simulink model "MotorPositionCntrl"  (R2020a)
settings: Solver=VariableStepAuto  StartTime=0.0  StopTime=10.0  FixedStep=0.01  RelTol=1e-3
undefined symbols (not defined in the file): b, J, K, L, R
settings Model: DataDictionary=MotorPositionCntrl.sldd  Creator=Admin  LastModifiedBy=Admin

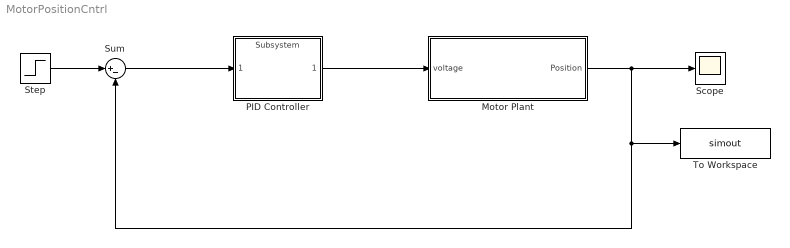
== system MotorPositionCntrl ==
  Motor Plant : Subsystem
  PID Controller : ModelReference  ModelNameDialog=Subsystem  ModelReferenceVersion=1.32
  Scope : Scope
  Step : Step  SampleTime=0
  Sum : Sum  Inputs=|+-
  To Workspace : ToWorkspace  VariableName=simout  SampleTime=-1
      settings: Save2DSignal=2-D array (concatenate along first dimension)
  wires:
  Motor Plant/1(Position) -> Sum/2, To Workspace/1, Scope/1
  Step/1 -> Sum/1
  Sum/1 -> PID Controller/1
  PID Controller/1 -> Motor Plant/1(voltage)

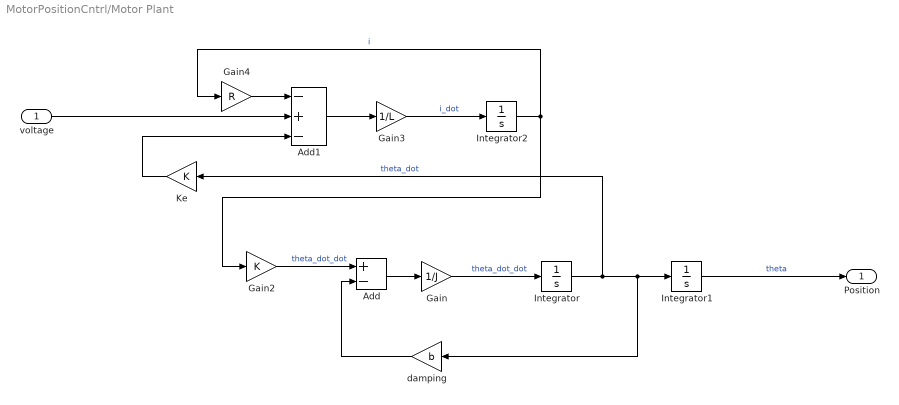
== system MotorPositionCntrl/Motor Plant ==
  voltage : Inport
  Add : Sum  Inputs=+-
  Add1 : Sum  Inputs=-+-
  Gain : Gain  Gain=1/J
  Gain2 : Gain  Gain=K
  Gain3 : Gain  Gain=1/L
  Gain4 : Gain  Gain=R
  Integrator : Integrator
  Integrator1 : Integrator
  Integrator2 : Integrator
  Ke : Gain  Gain=K
  damping : Gain  Gain=b
  Position : Outport
  wires:
  voltage/1 -> Add1/2
  damping/1 -> Add/2
  Gain/1 -> Integrator/1  "theta_dot_dot"
  Gain3/1 -> Integrator2/1  "i_dot"
  Integrator/1 -> Ke/1, damping/1, Integrator1/1  "theta_dot"
  Gain2/1 -> Add/1  "theta_dot_dot"
  Integrator2/1 -> Gain2/1, Gain4/1  "i"
  Gain4/1 -> Add1/1
  Add1/1 -> Gain3/1
  Ke/1 -> Add1/3
  Add/1 -> Gain/1
  Integrator1/1 -> Position/1  "theta"
